simulink model "aMedianFilter_2D_forHDL"  (Simulink 7.7)
settings: Solver=FixedStepDiscrete  SolverMode=SingleTasking  StartTime=0.0  StopTime=131*131  FixedStep=1  RelTol=1e-3
InitFcn:
  | wsize1 = uint32(3);
  | wsize2 = uint32(5);
  | wsize3 = uint32(7);
undefined symbols (not defined in the file): jet
libraries: simulink x2, vipsnks x2, vipsrcs x1
settings Model: Creator=kkintali  LastModifiedBy=kkintali  ExtModeAutoUpdateStatusClock=off
settings DataIOCC: SaveOutput=off  SignalLogging=off  SaveTime=off
settings OptimizationCC: BlockReduction=off  ConditionallyExecuteInputs=off  InlineParams=on  InitFltsAndDblsToZero=on  EfficientMapNaN2IntZero=off
settings DebuggingCC: AlgebraicLoopMsg=error  SingleTaskRateTransMsg=error  StrictBusMsg=Warning
settings HardwareCC: ProdHWDeviceType=ASIC/FPGA->ASIC/FPGA
settings SFSimCC: SimParseCustomCode=off

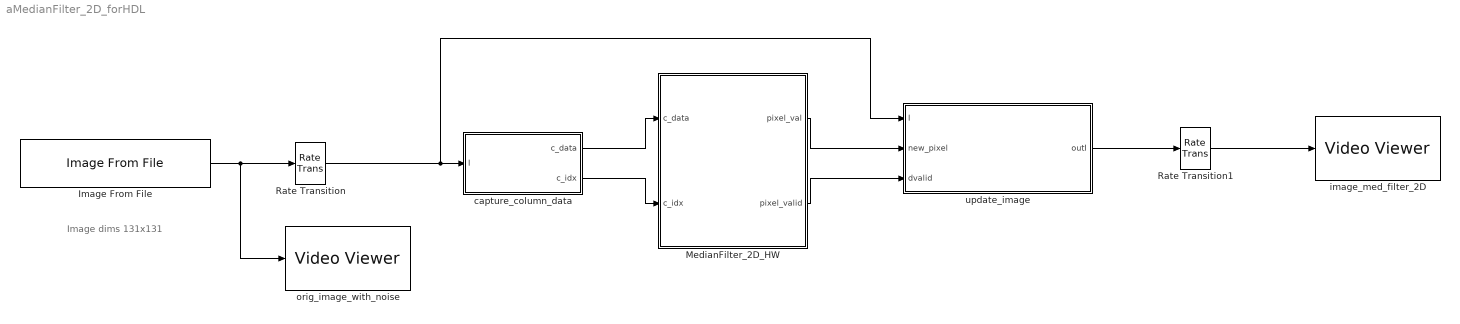
== system aMedianFilter_2D_forHDL ==
  note: Image dims
      |  131x131
  Image From File : vipsrcs/Image From File  Tag=vipblks_nd  SystemSampleTime=-1  FileName=pattern_noisy_002.tif  imagePorts=One multidimensional signal  Ts=131*131  ImageDataType=uint8  Signed=on  WordLength=16  sdImageDataType=uint(8)  FractionLengthMode=User-defined  FractionLength=15  OutPortLabels=R
  MedianFilter_2D_HW : Subsystem
  Rate Transition : RateTransition  Integrity=off  Deterministic=off  OutPortSampleTime=1
  Rate Transition1 : RateTransition  Integrity=off  OutPortSampleTime=131*131
  capture_column_data : Stateflow chart  TreatAsAtomicUnit=on
  image_med_filter_2D : vipsnks/Video Viewer  inputType=Obsolete7b  imagePorts=One multidimensional signal  useColorMap=off  colormapValue=jet(256);  specRange=off  minInputVal=0  maxInputVal=255  FigPos=[971 687 237 176]  AxisZoom=on  trueSizedOnce=on  OpenAtMdlStart=on
  orig_image_with_noise : vipsnks/Video Viewer  inputType=Obsolete7b  imagePorts=One multidimensional signal  useColorMap=off  colormapValue=jet(256);  specRange=off  minInputVal=0  maxInputVal=255  FigPos=[707 688 237 176]  AxisZoom=on  trueSizedOnce=on  OpenAtMdlStart=on
  update_image : Stateflow chart  TreatAsAtomicUnit=on
  wires:
  MedianFilter_2D_HW/1(pixel_val) -> update_image/2(new_pixel)
  MedianFilter_2D_HW/2(pixel_valid) -> update_image/3(dvalid)
  Rate Transition/1 -> capture_column_data/1(I), update_image/1(I)
  capture_column_data/1(c_data) -> MedianFilter_2D_HW/1(c_data)
  capture_column_data/2(c_idx) -> MedianFilter_2D_HW/2(c_idx)
  Rate Transition1/1 -> image_med_filter_2D/1
  update_image/1(outI) -> Rate Transition1/1
  Image From File/1 -> Rate Transition/1, orig_image_with_noise/1

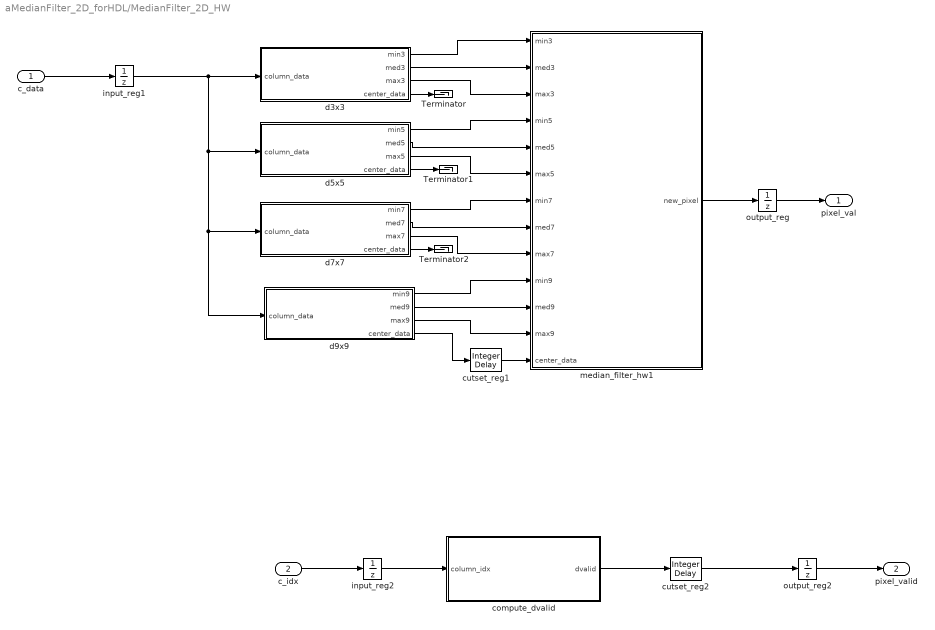
== system aMedianFilter_2D_forHDL/MedianFilter_2D_HW ==
  c_data : Inport
  c_idx : Inport  Port=2
  Terminator : Terminator
  Terminator1 : Terminator
  Terminator2 : Terminator
  compute_dvalid : Stateflow chart  TreatAsAtomicUnit=on
  cutset_reg1 : simulink/Discrete/Integer Delay  NumDelays=2  InputProcessing=Inherited  vinit=0.0  samptime=-1
  cutset_reg2 : simulink/Discrete/Integer Delay  NumDelays=2  InputProcessing=Inherited  vinit=0.0  samptime=-1
  d3x3 : Stateflow chart  TreatAsAtomicUnit=on
  d5x5 : Stateflow chart  TreatAsAtomicUnit=on
  d7x7 : Stateflow chart  TreatAsAtomicUnit=on
  d9x9 : Stateflow chart  TreatAsAtomicUnit=on
  input_reg1 : UnitDelay
  input_reg2 : UnitDelay
  median_filter_hw1 : Stateflow chart  TreatAsAtomicUnit=on
  output_reg : UnitDelay
  output_reg2 : UnitDelay
  pixel_val : Outport
  pixel_valid : Outport  Port=2
  wires:
  c_data/1 -> input_reg1/1
  c_idx/1 -> input_reg2/1
  compute_dvalid/1(dvalid) -> cutset_reg2/1
  median_filter_hw1/1(new_pixel) -> output_reg/1
  d3x3/4(center_data) -> Terminator/1
  d3x3/1(min3) -> median_filter_hw1/1(min3)
  d3x3/2(med3) -> median_filter_hw1/2(med3)
  d3x3/3(max3) -> median_filter_hw1/3(max3)
  d5x5/1(min5) -> median_filter_hw1/4(min5)
  d5x5/2(med5) -> median_filter_hw1/5(med5)
  d5x5/3(max5) -> median_filter_hw1/6(max5)
  d5x5/4(center_data) -> Terminator1/1
  d7x7/4(center_data) -> Terminator2/1
  d7x7/1(min7) -> median_filter_hw1/7(min7)
  d7x7/2(med7) -> median_filter_hw1/8(med7)
  d7x7/3(max7) -> median_filter_hw1/9(max7)
  d9x9/1(min9) -> median_filter_hw1/10(min9)
  d9x9/2(med9) -> median_filter_hw1/11(med9)
  d9x9/3(max9) -> median_filter_hw1/12(max9)
  d9x9/4(center_data) -> cutset_reg1/1
  cutset_reg1/1 -> median_filter_hw1/13(center_data)
  input_reg1/1 -> d3x3/1(column_data), d5x5/1(column_data), d7x7/1(column_data), d9x9/1(column_data)
  output_reg/1 -> pixel_val/1
  output_reg2/1 -> pixel_valid/1
  input_reg2/1 -> compute_dvalid/1(column_idx)
  cutset_reg2/1 -> output_reg2/1

== matlab function update_image ==
  data: I input double; new_pixel input double; dvalid input double; outI output double
function outI  = reconstruct_data(I, new_pixel, dvalid)

smax = 9;

% center pixel
cp = uint32(ceil(smax/2));

[nrows ncols] = size(I);

persistent newI;
if isempty(newI)
    newI = I;
end

persistent col_idx;
persistent row_idx;

if isempty(row_idx)
    row_idx = cp;
    col_idx = cp;
end

outI = newI;

if dvalid == true
    newI(row_idx, col_idx) = new_pixel;
    
    if (col_idx == ncols-cp+1)
        col_idx = cp;
        if (row_idx == nrows-cp+1)
            row_idx = cp;
        else
            row_idx = row_idx+1;
        end
    else
        col_idx = col_idx+1;
    end
end

== matlab function MedianFilter_2D_HW/d3x3 ==
  data: column_data input double; min3 output double; med3 output double; max3 output double; center_data output double
function [ min3, med3, max3, center_data] = d3x3(column_data)

smax = 9;

% storage for 9x9 buffer
persistent data;
if isempty(data)
    data = uint8(zeros(smax,smax));
end

w3 = -1:1;

% center pixel
cp = ceil(smax/2);

% compute region indices
r3 = cp+w3;

% get the region
d3x3  = data(r3, r3);

% get the centre pixel value
center_data = data(cp, cp);

% compute 2d median on 3x3 window 
% USE 1D filter for 3X3 window.
persistent min3_reg1 min3_reg2 med3_reg1 med3_reg2 max3_reg1 max3_reg2
if isempty(min3_reg1)
    min3_reg1 = uint8(0);
    min3_reg2 = uint8(0);
    med3_reg1 = uint8(0);
    med3_reg2 = uint8(0);
    max3_reg1 = uint8(0);
    max3_reg2 = uint8(0);
end
min3      = min3_reg2;
min3_reg2 = min3_reg1;
med3      = med3_reg2;
med3_reg2 = med3_reg1;
max3      = max3_reg2;
max3_reg2 = max3_reg1;
    
combine_d3x3 = d3x3(:)';
outbuf = get_median_1d(combine_d3x3);

numpixels = length(combine_d3x3);
max3_reg1 = outbuf(1);
med3_reg1 = outbuf(ceil(numpixels/2));
min3_reg1 = outbuf(numpixels);

% build the 9x9 buffer
data(:,2:smax) = data(:,1:smax-1);
data(:,1) = column_data;

end

== matlab function MedianFilter_2D_HW/d5x5 ==
  data: column_data input double; min5 output double; med5 output double; max5 output double; center_data output double
function [min5, med5, max5, center_data] = d5x5(column_data)

smax = 9;

% storage for 9x9 buffer
persistent data;
if isempty(data)
    data = uint8(zeros(smax,smax));
end

w5 = -2:2;

% center pixel
cp = ceil(smax/2);

% compute region indices
r5 = cp+w5;

% get the region
d5x5  = data(r5, r5);

% get the centre pixel value
center_data = data(cp, cp);

% compute 2d median on 5x5 window
[min5, med5, max5] = get_median_2d(d5x5);

% build the 9x9 buffer
data(:,2:smax) = data(:,1:smax-1);
data(:,1) = column_data;

end

% 2D median filter implementation 
% using two 1D median filters
% apply median filter on rows first followed by columns
% insert a delay to break long critical path
%
%   inbuf --> row_processor --> delay --> delay --> column_processor --> outbuf

function [min,med,max] = get_median_2d(inbuf)

[nrows ncols] = size(inbuf);

% two level register to store the median values computed from rows
persistent temp_buf1;
if isempty(temp_buf1)
    temp_buf1 = uint8(zeros(nrows,ncols));
end

persistent temp_buf2;
if isempty(temp_buf2)
	temp_buf2 = uint8(zeros(nrows,ncols));
end

outbuf = inbuf;

% compute median values of columns
for jj=coder.unroll(1:ncols)
    outbuf(:, jj) = get_median_1d(temp_buf2(:, jj)')';
end

temp_buf2 = temp_buf1;

% compute median values of rows
for ii=coder.unroll(1:nrows)
    temp_buf1(ii, :) = get_median_1d(inbuf(ii, :));
end


% pick min,med,max from outbuf
max = outbuf(1, 1);
med = outbuf(ceil(nrows/2), ceil(ncols/2));
min = outbuf(nrows, ncols);

end

== matlab function MedianFilter_2D_HW/d7x7 ==
  data: column_data input double; min7 output double; med7 output double; max7 output double; center_data output double
function [min7, med7, max7, center_data] = d7x7(column_data)

smax = 9;

% storage for 9x9 buffer
persistent data;
if isempty(data)
    data = uint8(zeros(smax,smax));
end

w7 = -3:3;

% center pixel
cp = ceil(smax/2);

% compute region indices
r7 = cp+w7;

% get the region
d7x7  = data(r7, r7);

% get the centre pixel value
center_data = data(cp, cp);

% compute 2d median on 7x7 window
[min7, med7, max7] = get_median_2d(d7x7);

% build the 9x9 buffer
data(:,2:smax) = data(:,1:smax-1);
data(:,1) = column_data;

end

% 2D median filter implementation 
% using two 1D median filters
% apply median filter on rows first followed by columns
% insert a delay to break long critical path
%
%   inbuf --> row_processor --> delay --> delay --> column_processor --> outbuf

function [min,med,max] = get_median_2d(inbuf)

[nrows ncols] = size(inbuf);

% two level register to store the median values computed from rows
persistent temp_buf1;
if isempty(temp_buf1)
    temp_buf1 = uint8(zeros(nrows,ncols));
end

persistent temp_buf2;
if isempty(temp_buf2)
	temp_buf2 = uint8(zeros(nrows,ncols));
end

outbuf = inbuf;

% compute median values of columns
for jj=eml.unroll(1:ncols)
    outbuf(:, jj) = get_median_1d(temp_buf2(:, jj)')';
end

temp_buf2 = temp_buf1;

% compute median values of rows
for ii=eml.unroll(1:nrows)
    temp_buf1(ii, :) = get_median_1d(inbuf(ii, :));
end


% pick min,med,max from outbuf
max = outbuf(1, 1);
med = outbuf(ceil(nrows/2), ceil(ncols/2));
min = outbuf(nrows, ncols);

end

== matlab function capture_column_data ==
  data: I input double; c_data output double; c_idx output double
function [c_data, c_idx] = get_data(I)
% return a 1x9 column at a time from the Image

smax = 9;

[nrows ncols] = size(I);

persistent col_idx;
persistent row_idx;

if isempty(row_idx)
    row_idx = uint32(1);
    col_idx = uint32(1);
end

c_idx = col_idx;

c_data = uint8(zeros(1,smax));

for ii=1:smax
    c_data(ii) = I(row_idx+ii-1, c_idx);
end


if (col_idx == ncols)
    col_idx = uint32(1);
    if (row_idx == nrows-smax+1)
        row_idx = uint32(1);
    else
        row_idx = row_idx+1;
    end
else
    col_idx = col_idx+1;
end

== matlab function MedianFilter_2D_HW/compute_dvalid ==
  data: dvalid output double; column_idx input double
function dvalid  = get_ctrl(column_idx)

% max size of the matrix buffered
smax = 9;

% we need to wait until 9 cycles for the buffer to fill up


persistent datavalid
if isempty(datavalid)
    datavalid = false;
end
dvalid = datavalid;
datavalid = (column_idx >= smax);

== matlab function MedianFilter_2D_HW/d9x9 ==
  data: column_data input double; min9 output double; med9 output double; max9 output double; center_data output double
function [min9, med9, max9, center_data] = d9x9(column_data)

smax = 9;

% storage for 9x9 buffer
persistent data;
if isempty(data)
    data = uint8(zeros(smax,smax));
end

w9 = -4:4;

% center pixel
cp = ceil(smax/2);

% compute region indices
r9 = cp+w9;

% get the region
d9x9  = data(r9, r9);

% get the centre pixel value
center_data = data(cp, cp);

% compute 2d median on 9x9 window
[min9, med9, max9] = get_median_2d(d9x9);

% build the 9x9 buffer
data(:,2:smax) = data(:,1:smax-1);
data(:,1) = column_data;

end

% 2D median filter implementation 
% using two 1D median filters
% apply median filter on rows first followed by columns
% insert a delay to break long critical path
%
% inbuf -> row_processor -> delay -> delay -> column_processor -> outbuf

function [min,med,max] = get_median_2d(inbuf)

[nrows ncols] = size(inbuf);

% two level register to store the median values computed from rows
persistent temp_buf1;
if isempty(temp_buf1)
    temp_buf1 = uint8(zeros(nrows,ncols));
end

persistent temp_buf2;
if isempty(temp_buf2)
	temp_buf2 = uint8(zeros(nrows,ncols));
end

outbuf = inbuf;

% compute median values of columns
for jj=coder.unroll(1:ncols)
    outbuf(:, jj) = get_median_1d(temp_buf2(:, jj)')';
end

temp_buf2 = temp_buf1;

% compute median values of rows
for ii=coder.unroll(1:nrows)
    temp_buf1(ii, :) = get_median_1d(inbuf(ii, :));
end


% pick min,med,max from outbuf
max = outbuf(1, 1);
med = outbuf(ceil(nrows/2), ceil(ncols/2));
min = outbuf(nrows, ncols);

end

== matlab function MedianFilter_2D_HW/median_filter_hw1 ==
  data: new_pixel output double; min3 input double; med3 input double; max3 input double; min5 input double; med5 input double; max5 input double; min7 input double; med7 input double; max7 input double; min9 input double; med9 input double; max9 input double; center_data input double
function new_pixel  = get_new_pixel(min3, med3, max3, ...
                                    min5, med5, max5, ...
                                    min7, med7, max7, ...
                                    min9, med9, max9, ...
                                    center_data)



if (med3 > min3 && med3 < max3)
    new_pixel = get_center_data(min3, med3, max3,center_data);
elseif (med5 > min5 && med5 < max5)
    new_pixel = get_center_data(min5, med5, max5,center_data);
elseif (med7 > min7 && med7 < max7)
    new_pixel = get_center_data(min7, med7, max7,center_data);
elseif (med9 > min9 && med9 < max9)
    new_pixel = get_center_data(min9, med9, max9,center_data);
else
    new_pixel = center_data;
end
